simulink model "simulation"  (R2021a)
settings: Solver=VariableStepAuto  StartTime=0.0  StopTime=150  RelTol=1e-3
settings Model: Creator=hanif  LastModifiedBy=hanif

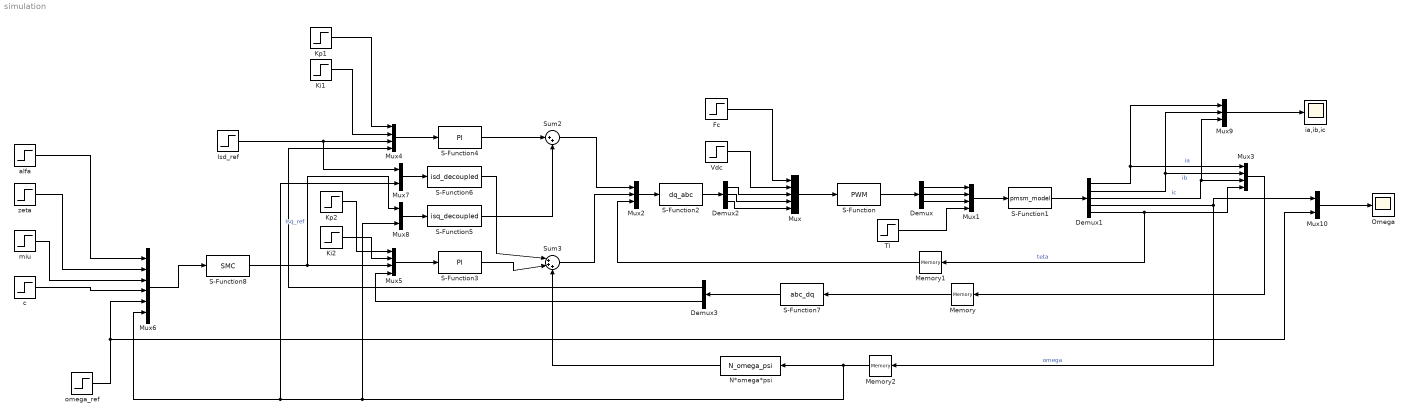
== system simulation ==
  Demux : Demux  Outputs=3
  Demux1 : Demux  Outputs=5
  Demux2 : Demux  Outputs=3
  Demux3 : Demux  Outputs=2
  Fc : Step  Time=0  After=500  SampleTime=0
  Isd_ref : Step  Time=0  After=0  SampleTime=0
  Ki1 : Step  Time=0  After=0.01  SampleTime=0
  Ki2 : Step  Time=0  After=0.01  SampleTime=0
  Kp1 : Step  Time=0  After=0.01  SampleTime=0
  Kp2 : Step  Time=0  After=0.01  SampleTime=0
  Memory : Memory
  Memory1 : Memory
  Memory2 : Memory
  Mux : Mux  Inputs=5
  Mux{1,3..5} (4 alike) : Mux
  Mux10 : Mux  Inputs=2
  Mux2 : Mux  Inputs=3
  Mux6 : Mux  Inputs=6
  Mux7 : Mux  Inputs=2
  Mux8 : Mux  Inputs=2
  Mux9 : Mux  Inputs=3
  N*omega*psi : S-Function  FunctionName=N_omega_psi  SFunctionDeploymentMode=off  EnableBusSupport=off
  Omega : Scope
  S-Function : S-Function  FunctionName=PWM  SFunctionDeploymentMode=off  EnableBusSupport=off
  S-Function1 : S-Function  FunctionName=pmsm_model  SFunctionDeploymentMode=off  EnableBusSupport=off
  S-Function2 : S-Function  FunctionName=dq_abc  SFunctionDeploymentMode=off  EnableBusSupport=off
  S-Function3 : S-Function  FunctionName=PI  SFunctionDeploymentMode=off  EnableBusSupport=off
  S-Function4 : S-Function  FunctionName=PI  SFunctionDeploymentMode=off  EnableBusSupport=off
  S-Function5 : S-Function  FunctionName=isq_decoupled  SFunctionDeploymentMode=off  EnableBusSupport=off
  S-Function6 : S-Function  FunctionName=isd_decoupled  SFunctionDeploymentMode=off  EnableBusSupport=off
  S-Function7 : S-Function  FunctionName=abc_dq  SFunctionDeploymentMode=off  EnableBusSupport=off
  S-Function8 : S-Function  FunctionName=SMC  SFunctionDeploymentMode=off  EnableBusSupport=off
  Sum2 : Sum  Inputs=|++
  Sum3 : Sum  Inputs=|+++
  Tl : Step  Time=0  After=0  SampleTime=0
  Vdc : Step  Time=0  After=1000  SampleTime=0
  alfa : Step  Time=0  After=60  SampleTime=0
  c : Step  Time=0  After=40  SampleTime=0
  ia,ib,ic : Scope
  miu : Step  Time=0  After=40  SampleTime=0
  omega_ref : Step  Time=50  Before=250  After=250  SampleTime=0
  zeta : Step  Time=0  After=100  SampleTime=0
  wires:
  Mux1/1 -> S-Function1/1
  S-Function1/1 -> Demux1/1
  Demux/1 -> Mux1/1
  Demux/2 -> Mux1/2
  Demux/3 -> Mux1/3
  S-Function/1 -> Demux/1
  S-Function2/1 -> Demux2/1
  Mux/1 -> S-Function/1
  S-Function4/1 -> Sum2/1
  S-Function3/1 -> Sum3/2
  S-Function6/1 -> Sum3/1
  S-Function5/1 -> Sum2/2
  Mux2/1 -> S-Function2/1
  Sum2/1 -> Mux2/1
  Sum3/1 -> Mux2/2
  Demux1/1 -> Mux9/1, Mux3/1  "ia"
  Demux1/2 -> Mux9/2, Mux3/2  "ib"
  Demux1/3 -> Mux9/3, Mux3/3  "ic"
  Memory/1 -> S-Function7/1
  S-Function7/1 -> Demux3/1
  Memory1/1 -> Mux2/3
  Demux1/5 -> Memory1/1, Mux3/4  "teta"
  Mux3/1 -> Memory/1
  Demux1/4 -> Mux10/1, Memory2/1  "omega"
  Memory2/1 -> Mux6/6, Mux7/2, Mux8/2, N*omega*psi/1
  N*omega*psi/1 -> Sum3/3
  Mux4/1 -> S-Function4/1
  Mux5/1 -> S-Function3/1
  Kp1/1 -> Mux4/1
  Ki1/1 -> Mux4/2
  Kp2/1 -> Mux5/1
  Ki2/1 -> Mux5/2
  Isd_ref/1 -> Mux7/1, Mux4/3
  Mux6/1 -> S-Function8/1
  S-Function8/1 -> Mux5/3, Mux8/1  "Isq_ref"
  Demux3/1 -> Mux4/4
  Demux3/2 -> Mux5/4
  Fc/1 -> Mux/1
  Vdc/1 -> Mux/2
  Demux2/1 -> Mux/3
  Demux2/2 -> Mux/4
  Demux2/3 -> Mux/5
  Mux7/1 -> S-Function6/1
  Mux8/1 -> S-Function5/1
  Mux9/1 -> ia,ib,ic/1
  Tl/1 -> Mux1/4
  omega_ref/1 -> Mux6/5, Mux10/2
  ? -> ?
  Mux10/1 -> Omega/1
  alfa/1 -> Mux6/1
  zeta/1 -> Mux6/2
  miu/1 -> Mux6/3
  c/1 -> Mux6/4
